simulink model "magball2018"  (R2022a)
settings: Solver=FixedStepAuto  StartTime=0.0  StopTime=50  FixedStep=50e-6  RelTol=1e-3
values from neighbouring files (symbols this model uses):
  K = -place(A, B, poles)    [linearize.m]
  T = 0.05    [linearize.m]
settings Model: Creator=vishn  LastModifiedBy=user
settings SolverCC: AlgebraicLoopSolver=TrustRegion
settings DebuggingCC: UnconnectedInputMsg=warning  UnconnectedOutputMsg=warning  UnconnectedLineMsg=warning  ArithmeticOperatorsInVariantConditions=warning
settings SFSimCC: CustomCodeUndefinedFunction=UseInterfaceOnly

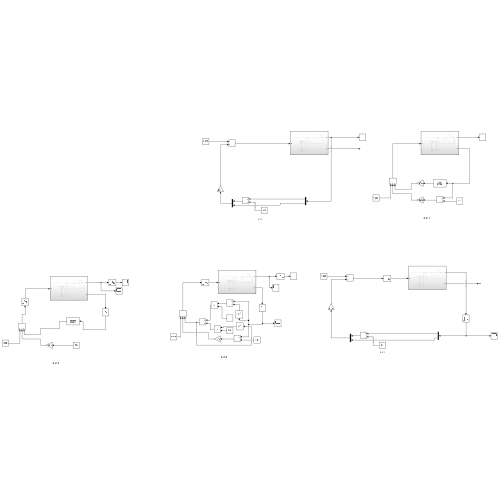
[thumbnail: Simulink's stored preview of the top-level diagram]
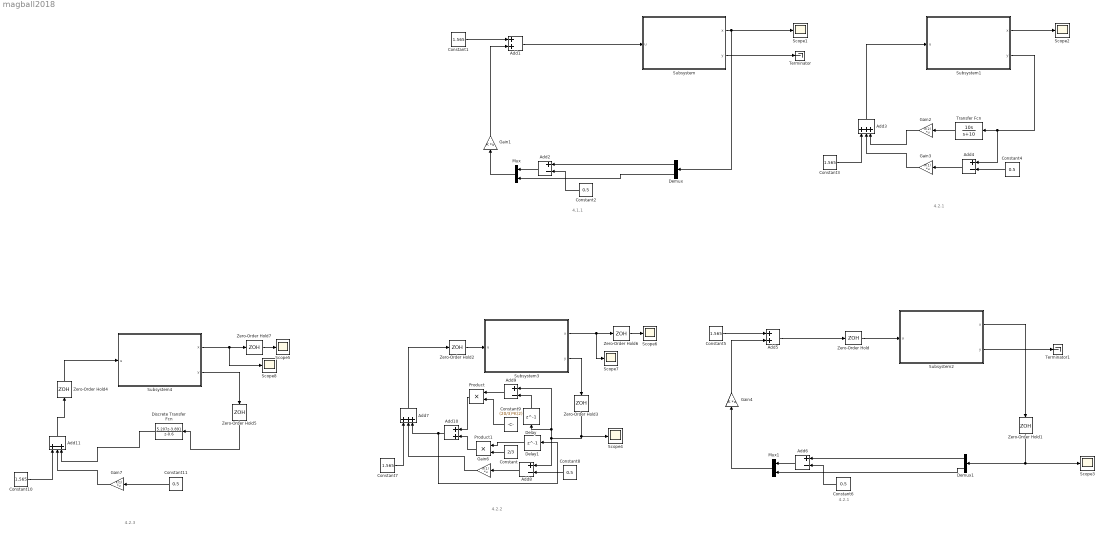
== system magball2018 ==
  note: 4.2.1
  note: 4.1.1
  note: 4.2.1
  note: 4.2.2
  note: 4.2.3
  Add1 : Sum
  Add10 : Sum
  Add11 : Sum  Inputs=+-+
  Add{2,4,6,8..9} (5 alike) : Sum  Inputs=+-
  Add3 : Sum  Inputs=+++
  Add5 : Sum
  Add7 : Sum  Inputs=+++
  Constant : Constant  Value=2/3
  Constant{1,3,5,7,10} (5 alike) : Constant  Value=1.565
  Constant{2,4,6,8,11} (5 alike) : Constant  Value=0.5
  Constant9 : Constant  Value=(20/3)*K(2)
  Delay : Delay  DelayLength=1
  Delay1 : Delay  DelayLength=1
  Demux : Demux  Outputs=2
  Demux1 : Demux  Outputs=2
  Discrete Transfer Fcn : DiscreteTransferFcn  Numerator=[5.207 , -3.891]  Denominator=[1 -0.6]
  Gain1 : Gain  Gain=K  Multiplication=Matrix(K*u)
  Gain2 : Gain  Gain=K(2)  Multiplication=Matrix(K*u)
  Gain3 : Gain  Gain=K(1)  Multiplication=Matrix(K*u)
  Gain4 : Gain  Gain=K  Multiplication=Matrix(K*u)
  Gain6 : Gain  Gain=K(1)  Multiplication=Matrix(K*u)
  Gain7 : Gain  Gain=K(1)  Multiplication=Matrix(K*u)
  Mux : Mux  Inputs=2
  Mux1 : Mux  Inputs=2
  Product : Product
  Product1 : Product
  Scope{1..8} (8 alike) : Scope
  Subsystem : Subsystem
  Subsystem1 : Subsystem
  Subsystem2 : Subsystem
  Subsystem3 : Subsystem
  Subsystem4 : Subsystem
  Terminator : Terminator
  Terminator1 : Terminator
  Transfer Fcn : TransferFcn  Numerator=[10 0]  Denominator=[1 10]
  Zero-Order Hold{,1..7} (8 alike) : ZeroOrderHold  SampleTime=T
  wires:
  Constant1/1 -> Add1/1
  Constant2/1 -> Add2/2
  Add2/1 -> Mux/1
  Mux/1 -> Gain1/1
  Gain1/1 -> Add1/2
  Add1/1 -> Subsystem/1("u ")
  Subsystem/1(x) -> Scope1/1, Demux/1
  Demux/1 -> Add2/1
  Demux/2 -> Mux/2
  Subsystem/2(y) -> Terminator/1
  Constant3/1 -> Add3/1
  Subsystem1/2(y) -> Add4/1, Transfer Fcn/1
  Transfer Fcn/1 -> Gain2/1
  Constant4/1 -> Add4/2
  Add4/1 -> Gain3/1
  Gain2/1 -> Add3/3
  Gain3/1 -> Add3/2
  Add3/1 -> Subsystem1/1("u ")
  Subsystem1/1(x) -> Scope2/1
  Constant5/1 -> Add5/1
  Mux1/1 -> Gain4/1
  Constant6/1 -> Add6/2
  Demux1/2 -> Mux1/2
  Subsystem2/1(x) -> Zero-Order Hold1/1
  Demux1/1 -> Add6/1
  Subsystem2/2(y) -> Terminator1/1
  Add6/1 -> Mux1/1
  Gain4/1 -> Add5/2
  Add5/1 -> Zero-Order Hold/1
  Zero-Order Hold/1 -> Subsystem2/1("u ")
  Zero-Order Hold1/1 -> Scope3/1, Demux1/1
  Gain6/1 -> Add7/2
  Constant7/1 -> Add7/1
  Constant8/1 -> Add8/2
  Add8/1 -> Gain6/1
  Subsystem3/1(x) -> Scope7/1, Zero-Order Hold6/1
  Zero-Order Hold2/1 -> Subsystem3/1("u ")
  Add7/1 -> Zero-Order Hold2/1
  Subsystem3/2(y) -> Zero-Order Hold3/1
  Zero-Order Hold3/1 -> Add9/1, Delay/1, Add8/1, Scope4/1
  Delay/1 -> Add9/2
  Add9/1 -> Product/1
  Product/1 -> Add10/1
  Add10/1 -> Delay1/1, Add7/3
  Constant/1 -> Product1/2
  Delay1/1 -> Product1/1
  Product1/1 -> Add10/2
  Constant9/1 -> Product/2
  Gain7/1 -> Add11/2
  Discrete Transfer Fcn/1 -> Add11/3
  Constant10/1 -> Add11/1
  Add11/1 -> Zero-Order Hold4/1
  Zero-Order Hold4/1 -> Subsystem4/1("u ")
  Subsystem4/2(y) -> Zero-Order Hold5/1
  Zero-Order Hold5/1 -> Discrete Transfer Fcn/1
  Constant11/1 -> Gain7/1
  Zero-Order Hold6/1 -> Scope6/1
  Zero-Order Hold7/1 -> Scope5/1
  Subsystem4/1(x) -> Scope8/1, Zero-Order Hold7/1

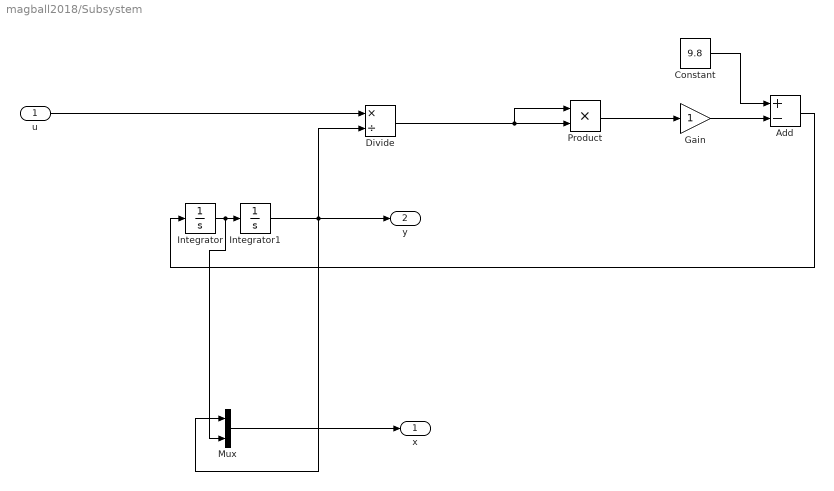
== system magball2018/Subsystem ==
  "u " : Inport
  Add : Sum  Inputs=+-
  Constant : Constant  Value=9.8
  Divide : Product  Inputs=*/
  Gain : Gain
  Integrator : Integrator  InitialCondition=0.5
  Integrator1 : Integrator  InitialCondition=1.3
  Mux : Mux  Inputs=2
  Product : Product
  x : Outport  VectorParamsAs1DForOutWhenUnconnected=off
  y : Outport  Port=2  VectorParamsAs1DForOutWhenUnconnected=off
  wires:
  "u "/1 -> Divide/1
  Integrator1/1 -> Mux/1, y/1, Divide/2
  Product/1 -> Gain/1
  Gain/1 -> Add/2
  Integrator/1 -> Mux/2, Integrator1/1
  Constant/1 -> Add/1
  Divide/1 -> Product/1, Product/2
  Add/1 -> Integrator/1
  Mux/1 -> x/1

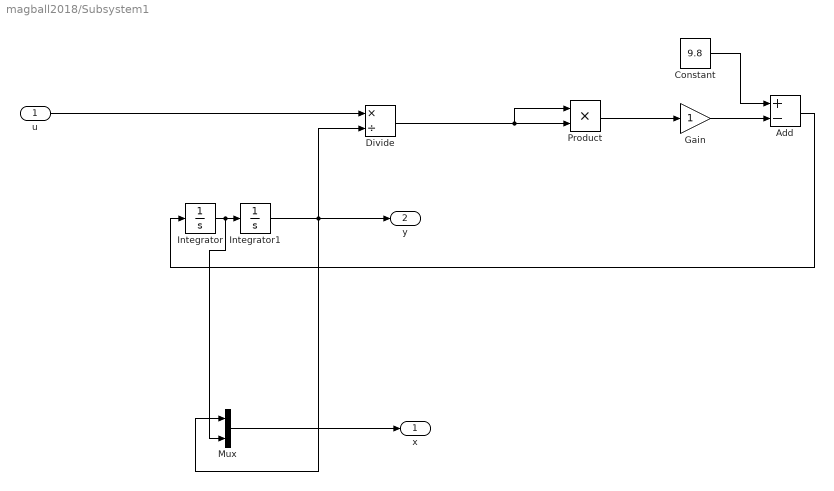
== system magball2018/Subsystem1 ==
  "u " : Inport
  Add : Sum  Inputs=+-
  Constant : Constant  Value=9.8
  Divide : Product  Inputs=*/
  Gain : Gain
  Integrator : Integrator  InitialCondition=0.5
  Integrator1 : Integrator  InitialCondition=1.3
  Mux : Mux  Inputs=2
  Product : Product
  x : Outport  VectorParamsAs1DForOutWhenUnconnected=off
  y : Outport  Port=2  VectorParamsAs1DForOutWhenUnconnected=off
  wires:
  "u "/1 -> Divide/1
  Integrator1/1 -> Mux/1, y/1, Divide/2
  Product/1 -> Gain/1
  Gain/1 -> Add/2
  Integrator/1 -> Mux/2, Integrator1/1
  Constant/1 -> Add/1
  Divide/1 -> Product/1, Product/2
  Add/1 -> Integrator/1
  Mux/1 -> x/1

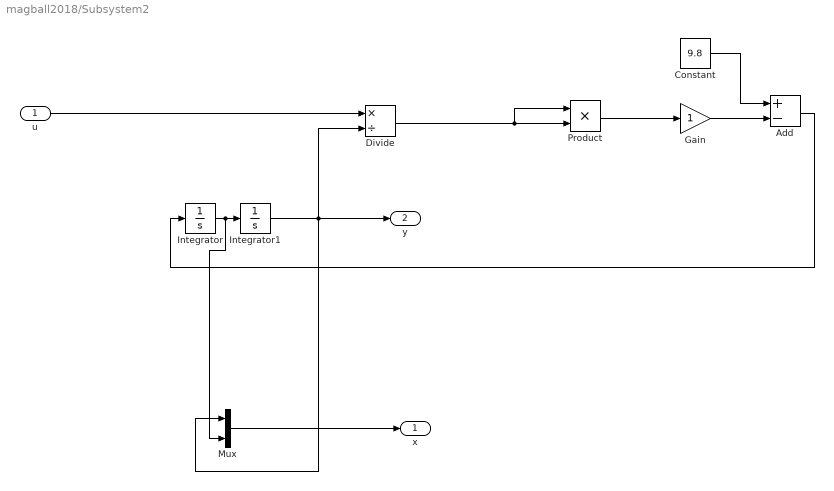
== system magball2018/Subsystem2 ==
  "u " : Inport
  Add : Sum  Inputs=+-
  Constant : Constant  Value=9.8
  Divide : Product  Inputs=*/
  Gain : Gain
  Integrator : Integrator  InitialCondition=0.5
  Integrator1 : Integrator  InitialCondition=1.3
  Mux : Mux  Inputs=2
  Product : Product
  x : Outport  VectorParamsAs1DForOutWhenUnconnected=off
  y : Outport  Port=2  VectorParamsAs1DForOutWhenUnconnected=off
  wires:
  "u "/1 -> Divide/1
  Integrator1/1 -> Mux/1, y/1, Divide/2
  Product/1 -> Gain/1
  Gain/1 -> Add/2
  Integrator/1 -> Mux/2, Integrator1/1
  Constant/1 -> Add/1
  Divide/1 -> Product/1, Product/2
  Add/1 -> Integrator/1
  Mux/1 -> x/1

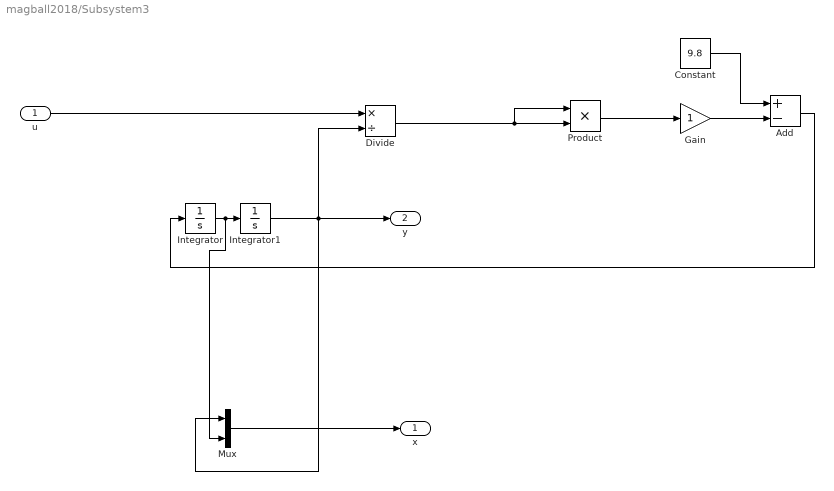
== system magball2018/Subsystem3 ==
  "u " : Inport
  Add : Sum  Inputs=+-
  Constant : Constant  Value=9.8
  Divide : Product  Inputs=*/
  Gain : Gain
  Integrator : Integrator  InitialCondition=0.5
  Integrator1 : Integrator  InitialCondition=1.3
  Mux : Mux  Inputs=2
  Product : Product
  x : Outport  VectorParamsAs1DForOutWhenUnconnected=off
  y : Outport  Port=2  VectorParamsAs1DForOutWhenUnconnected=off
  wires:
  "u "/1 -> Divide/1
  Integrator1/1 -> Mux/1, y/1, Divide/2
  Product/1 -> Gain/1
  Gain/1 -> Add/2
  Integrator/1 -> Mux/2, Integrator1/1
  Constant/1 -> Add/1
  Divide/1 -> Product/1, Product/2
  Add/1 -> Integrator/1
  Mux/1 -> x/1

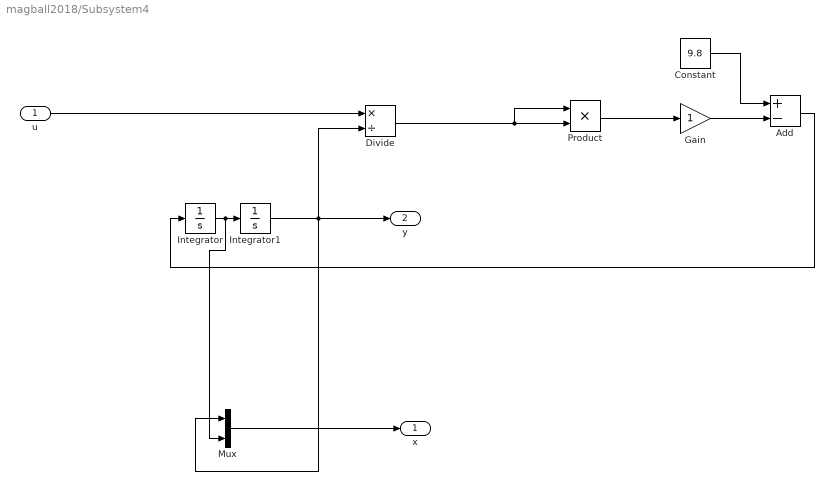
== system magball2018/Subsystem4 ==
  "u " : Inport
  Add : Sum  Inputs=+-
  Constant : Constant  Value=9.8
  Divide : Product  Inputs=*/
  Gain : Gain
  Integrator : Integrator  InitialCondition=0.5
  Integrator1 : Integrator  InitialCondition=1.3
  Mux : Mux  Inputs=2
  Product : Product
  x : Outport  VectorParamsAs1DForOutWhenUnconnected=off
  y : Outport  Port=2  VectorParamsAs1DForOutWhenUnconnected=off
  wires:
  "u "/1 -> Divide/1
  Integrator1/1 -> Mux/1, y/1, Divide/2
  Product/1 -> Gain/1
  Gain/1 -> Add/2
  Integrator/1 -> Mux/2, Integrator1/1
  Constant/1 -> Add/1
  Divide/1 -> Product/1, Product/2
  Add/1 -> Integrator/1
  Mux/1 -> x/1
